simulink model "Steering_Sensor_Finn"  (R2025b)
settings: Solver=FixedStepAuto  StartTime=0.0  StopTime=10.0  FixedStep=0.001  RelTol=1e-3
undefined symbols (not defined in the file): k_fehler
libraries: simulink x1
settings Model: NumberOfSteps=15  Creator=finneinhoff  LastModifiedBy=finneinhoff

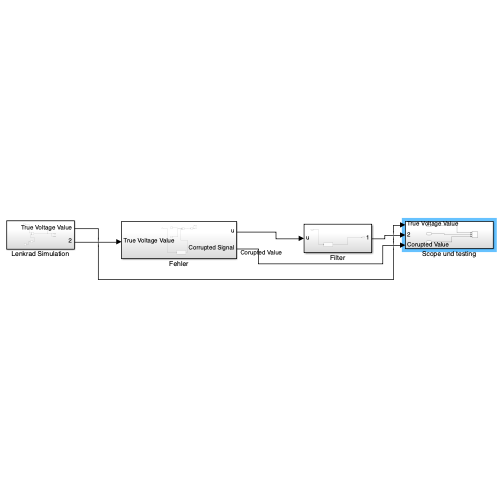
[thumbnail: Simulink's stored preview of the top-level diagram]
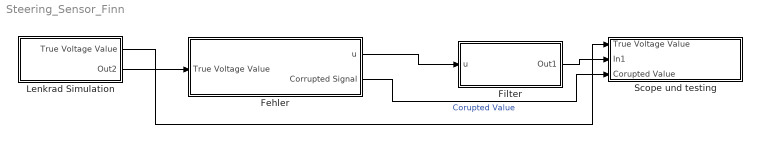
== system Steering_Sensor_Finn ==
  Fehler : Subsystem
  Filter : Subsystem
  Lenkrad Simulation : Subsystem
  Scope und testing : Subsystem
  wires:
  Fehler/2(Corrupted Signal) -> Scope und testing/3(Corupted Value)  "Corupted Value"
  Filter/1(Out1) -> Scope und testing/2(In1)
  Lenkrad Simulation/1(True Voltage Value) -> Scope und testing/1(True Voltage Value)
  Lenkrad Simulation/2(Out2) -> Fehler/1(True Voltage Value)
  Fehler/1(u) -> Filter/1(u)

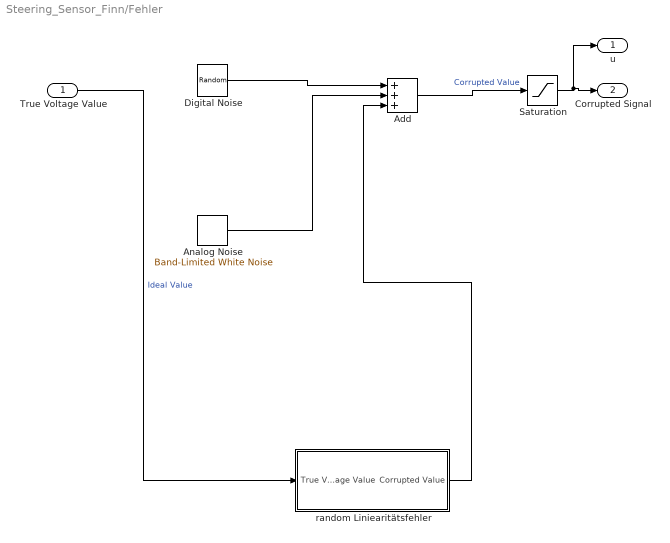
== system Steering_Sensor_Finn/Fehler ==
  True Voltage Value : Inport
  Add : Sum  Inputs=+++
  Analog Noise : simulink/Sources/Band-Limited White Noise  Cov=[1]  Ts=1  seed=23341
  Digital Noise : UniformRandomNumber  SampleTime=0.1
  Saturation : Saturate  UpperLimit=4.75  LowerLimit=0.25
  random Liniearitätsfehler : Subsystem
  u : Outport
  Corrupted Signal : Outport  Port=2
  wires:
  Saturation/1 -> Corrupted Signal/1, u/1
  Analog Noise/1 -> Add/2
  True Voltage Value/1 -> random Liniearitätsfehler/1(True Voltage Value)  "Ideal Value"
  random Liniearitätsfehler/1(Corrupted Value) -> Add/3
  Add/1 -> Saturation/1  "Corrupted Value"
  Digital Noise/1 -> Add/1

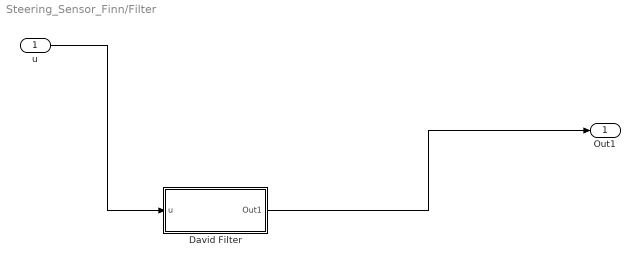
== system Steering_Sensor_Finn/Filter ==
  u : Inport
  David Filter : Subsystem
  Out1 : Outport
  wires:
  u/1 -> David Filter/1(u)
  David Filter/1(Out1) -> Out1/1

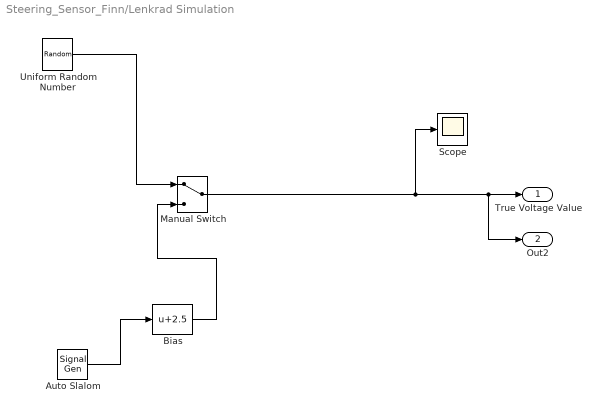
== system Steering_Sensor_Finn/Lenkrad Simulation ==
  Auto Slalom : SignalGenerator  Amplitude=2.25  Frequency=2  Units=rad/sec
  Bias : Bias  Bias=2.5  SaturateOnIntegerOverflow=off
  Manual Switch : ManualSwitch
  Scope : Scope
      settings: ActiveDisplayYMinimum=-0.27322298923890231  ActiveDisplayYMaximum=5.3054252826517567
  Uniform Random Number : UniformRandomNumber  Minimum=0.25  Maximum=4.75  SampleTime=0.5
  True Voltage Value : Outport
  Out2 : Outport  Port=2
  wires:
  Uniform Random Number/1 -> Manual Switch/1
  Auto Slalom/1 -> Bias/1
  Bias/1 -> Manual Switch/2
  Manual Switch/1 -> Scope/1, Out2/1, True Voltage Value/1

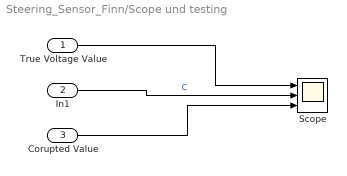
== system Steering_Sensor_Finn/Scope und testing ==
  True Voltage Value : Inport
  In1 : Inport  Port=2
  Corupted Value : Inport  Port=3
  Scope : Scope  NumInputPorts=3
      settings: ActiveDisplayYMinimum=-0.31249999999999989  ActiveDisplayYMaximum=5.3125
  wires:
  In1/1 -> Scope/2  "C"
  True Voltage Value/1 -> Scope/1
  Corupted Value/1 -> Scope/3

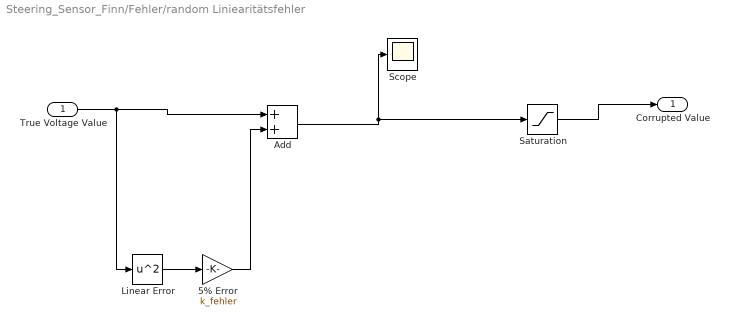
== system Steering_Sensor_Finn/Fehler/random Liniearitätsfehler ==
  True Voltage Value : Inport
  5% Error : Gain  Gain=k_fehler
  Add : Sum
  Linear Error : Math  Operator=square
  Saturation : Saturate  UpperLimit=4.75  LowerLimit=0.25
  Scope : Scope
      settings: ActiveDisplayYMinimum=-1  ActiveDisplayYMaximum=1  DataLoggingVariableName=ScopeData3
  Corrupted Value : Outport
  wires:
  True Voltage Value/1 -> Add/1, Linear Error/1
  Linear Error/1 -> 5% Error/1
  5% Error/1 -> Add/2
  Add/1 -> Scope/1, Saturation/1
  Saturation/1 -> Corrupted Value/1

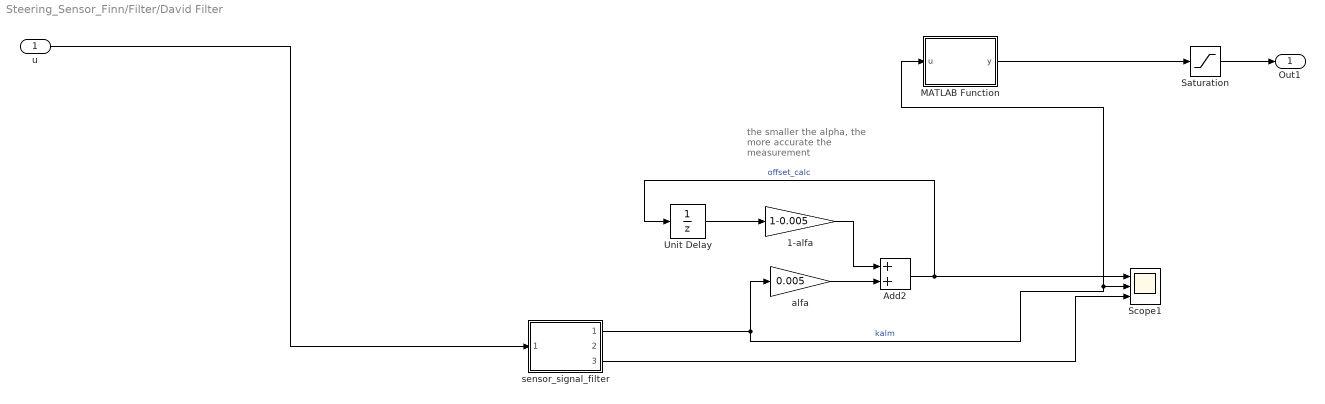
== system Steering_Sensor_Finn/Filter/David Filter ==
  note: the smaller the alpha, the more accurate the measurement
  u : Inport
  1-alfa : Gain  Gain=1-0.005
  Add2 : Sum
  MATLAB Function : MATLAB Function  TreatAsAtomicUnit=on
  Saturation : Saturate  UpperLimit=4.75  LowerLimit=0.25
  Scope1 : Scope  NumInputPorts=3
      settings: ActiveDisplayYMinimum=-0.61883444283566291  ActiveDisplayYMaximum=8.0096427868055873  DataLoggingVariableName=ScopeData4
  Unit Delay : UnitDelay  SampleTime=-1  HasFrameUpgradeWarning=on
  alfa : Gain  Gain=0.005
  sensor_signal_filter : MATLAB Function  TreatAsAtomicUnit=on
  Out1 : Outport
  wires:
  u/1 -> sensor_signal_filter/1(u_meas)
  Unit Delay/1 -> 1-alfa/1
  Add2/1 -> Unit Delay/1, Scope1/1  "offset_calc"
  sensor_signal_filter/1(pos_filtered) -> MATLAB Function/1(u), Scope1/2, alfa/1  "kalm"
  alfa/1 -> Add2/2
  1-alfa/1 -> Add2/1
  Saturation/1 -> Out1/1
  MATLAB Function/1(y) -> Saturation/1
  sensor_signal_filter/3(status_flag) -> Scope1/3

== matlab function Steering_Sensor_Finn/Filter/David Filter/MATLAB Function ==
  settings: updateMethod=DISCRETE
  data: u input; y output
function y = fcn(u)
    % Diese Funktion glättet den berechneten Offset.
    
    persistent x_est P first_run
    
    if isempty(first_run)
        x_est = u;
        P = 1.0;
        first_run = 0;
    end
    
    % --- TUNING ---
    % Wir machen Q etwas größer als vorher, damit der Offset nicht "einschläft",
    % falls sich die Temperatur o.ä. ändert.
    Q = 1e-4; 
    
    % R lassen wir hoch, damit das Ergebnis sehr stabil (glatt) ist.
    R = 5; 
   
    % Kalman Algorithmus
    P_pred = P + Q;
    K = P_pred / (P_pred + R);
    
    x_est = x_est + K * (u - x_est);
    P = (1 - K) * P_pred;
    
    y = x_est;
end

== matlab function Steering_Sensor_Finn/Filter/David Filter/sensor_signal_filter ==
  settings: updateMethod=DISCRETE
  data: u_meas input; pos_filtered output; vel_est output; status_flag output
function [pos_filtered, vel_est, status_flag] = KalmanFilter_Pro(u_meas)
%#codegen
% ROBUST KALMAN FILTER (Constant Velocity Model)
% Features: Outlier Rejection (Gating), Coasting, Numerical Stability
%
% Inputs:
%   u_meas: Rohes Sensorsignal
% Outputs:
%   pos_filtered: Gefilterte Position (Das Signal, das du willst)
%   vel_est: Geschätzte Geschwindigkeit (nützlich für andere Regler)
%   status_flag: 0=OK, 1=Coasting(No Data), 2=Outlier Rejected

% --- PERSISTENT MEMORY (Zustandsspeicher) ---
persistent x P          % Zustand [Pos; Vel] und Kovarianz
persistent first_run    % Initialisierungs-Flag
persistent outlier_cnt  % Zähler für aufeinanderfolgende Ausreißer

% --- KONFIGURATION (TUNING) ---
DT = 0.001;              % Sample Time (MUSS EXAKT STIMMEN!)

% Physik-Rauschen (Process Noise Q):
% Wie sehr darf sich die Geschwindigkeit pro Schritt ändern?
% Kleiner = Träger/Glatter. Größer = Aggressiver/Schneller.
SIGMA_ACCEL = 100.0;      
Q = [0.25*DT^4, 0.5*DT^3; 0.5*DT^3, DT^2] * SIGMA_ACCEL^2;

% Sensor-Rauschen (Measurement Noise R):
% Standardabweichung des Sensors (in Volt/Einheit).
% Erhöhe das, um das "Gezappel" zu glätten.
R_VAL = 2.0;            
R = R_VAL^2;            

% Gating Threshold (Chi-Square Test):
% 95% Konfidenz = 3.84, 99% = 6.63. 
% Ein Wert von 9.0 ist sehr robust (3-Sigma).
GATE_THRESH = 100.0;      

% Safety: Nach wie vielen ignorierten "Outliers" in Folge glauben wir dem
% Sensor trotzdem wieder? (Verhindert ewiges Wegdriften)
MAX_CONSECUTIVE_OUTLIERS = 10; 

% --- INITIALISIERUNG ---
if isempty(first_run)
    % Startzustand: Wir nehmen den ersten Messwert als Wahrheit
    if isnan(u_meas)
        x = [0; 0]; % Fallback falls Startwert NaN
    else
        x = [u_meas; 0];
    end
    
    % Initiale Unsicherheit (wir sind uns anfangs unsicher bei der Geschw.)
    P = [R_VAL, 0; 0, 100]; 
    
    outlier_cnt = 0;
    first_run = 0;
end

% --- SYSTEM MATRIZEN ---
% State Transition Matrix (Physik: x_neu = x_alt + v*t)
A = [1, DT; 0, 1];
% Measurement Matrix (Wir messen nur Position)
H = [1, 0];
I = eye(2); 

% ---------------------------------------------------------
% SCHRITT 1: PREDICT (Zeit-Update)
% "Wo müsste das System physikalisch jetzt sein?"
% ---------------------------------------------------------
x_pred = A * x;
P_pred = A * P * A' + Q;

% ---------------------------------------------------------
% SCHRITT 2: GATING & UPDATE (Mess-Update)
% ---------------------------------------------------------

% Prüfen: Ist Eingangssignal valide (kein NaN)?
if ~isnan(u_meas)
    
    % 1. Innovation (Residuum): Unterschied Messung <-> Vorhersage
    y_res = u_meas - (H * x_pred);
    
    % 2. Innovations-Kovarianz (Gesamtunsicherheit S)
    S = H * P_pred * H' + R;
    
    % 3. Mahalanobis Distanz (Quadriert)
    % Das ist der "Professionalitäts-Check": Ist der Abstand statistisch signifikant?
    % (Abweichung)^2 / Unsicherheit
    nis = (y_res^2) / S;
    
    % 4. Logik-Entscheidung
    is_outlier = (nis > GATE_THRESH);
    
    % Force Update falls wir zu lange "blind" geflogen sind (Recovery)
    if outlier_cnt >= MAX_CONSECUTIVE_OUTLIERS
        is_outlier = false; 
    end
    
    if is_outlier
        % --- FALL A: AUSREISSER (Reject) ---
        % Wir ignorieren die Messung und vertrauen voll der Physik.
        % Der Zustand wird nur durch die Prediction aktualisiert.
        x = x_pred;
        P = P_pred;
        
        outlier_cnt = outlier_cnt + 1;
        status_flag = 2; % Debug Code "Outlier"
        
    else
        % --- FALL B: GÜLTIGE MESSUNG (Update) ---
        % Kalman Gain berechnen
        K = P_pred * H' / S;
        
        % Zustand korrigieren (Optimal Fusion)
        x = x_pred + K * y_res;
        
        % Kovarianz updaten (Joseph Form für numerische Stabilität wäre besser,
        % aber die einfache Form reicht hier meistens)
        P = (I - K * H) * P_pred;
        
        outlier_cnt = 0; % Counter reset
        status_flag = 0; % Debug Code "OK"
    end
    
else
    % --- FALL C: SIGNAL LOST (NaN input) ---
    % Wir fliegen blind auf Basis des Physik-Modells weiter (Coasting)
    x = x_pred;
    P = P_pred;
    status_flag = 1; % Debug Code "Coasting"
end

% --- SCHRITT 3: NUMERISCHE SICHERUNG ---
% Erzwinge Symmetrie der Matrix (verhindert komplexe Abstürze nach Stunden)
P = 0.5 * (P + P');

% --- OUTPUT ---
pos_filtered = x(1);
vel_est = x(2);

end
